simulink model "week2pro4"  (R2020b)
settings: Solver=VariableStepAuto  StartTime=0.0  StopTime=10.0  RelTol=1e-3
model workspace (MAT data in the model file):
  J = 3.224e-06
  K = 0.0274
  L = 2.75e-06
  R = 4
  b = 3.2577e-06
  kd = 0.14068535322
  ki = 523.295635458
  kp = 17.35894986
settings Model: Creator=admin  LastModifiedBy=admin

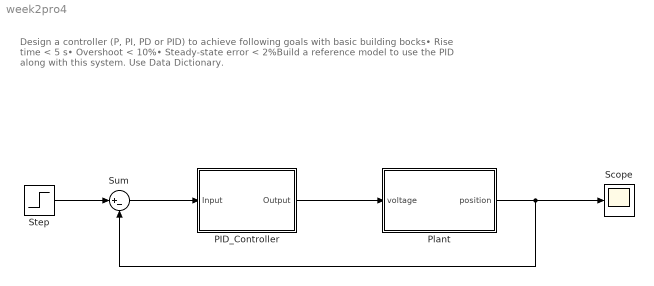
== system week2pro4 ==
  note: Design a controller (P, PI, PD or PID) to achieve following goals with basic building bocks• Rise time < 5 s• Overshoot < 10%• Steady-state error < 2%Build a reference model to use the PID along with this system. Use Data Dictionary.
  PID_Controller : Subsystem
  Plant : Subsystem
  Scope : Scope
  Step : Step  SampleTime=0
  Sum : Sum  Inputs=|+-
  wires:
  PID_Controller/1(Output) -> Plant/1(voltage)
  Sum/1 -> PID_Controller/1(Input)
  Step/1 -> Sum/1
  Plant/1(position) -> Sum/2, Scope/1

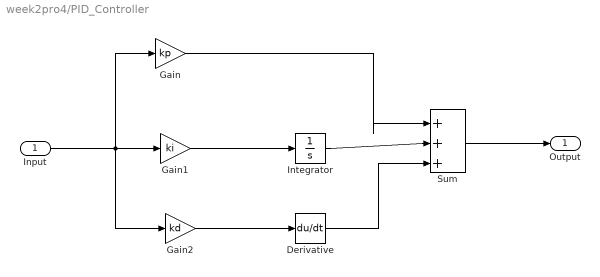
== system week2pro4/PID_Controller ==
  Input : Inport
  Derivative : Derivative
  Gain : Gain  Gain=kp
  Gain1 : Gain  Gain=ki
  Gain2 : Gain  Gain=kd
  Integrator : Integrator
  Sum : Sum  Inputs=|+++
  Output : Outport
  wires:
  Gain1/1 -> Integrator/1
  Input/1 -> Gain2/1, Gain/1, Gain1/1
  Derivative/1 -> Sum/3
  Gain/1 -> Sum/1
  Sum/1 -> Output/1
  Integrator/1 -> Sum/2
  Gain2/1 -> Derivative/1

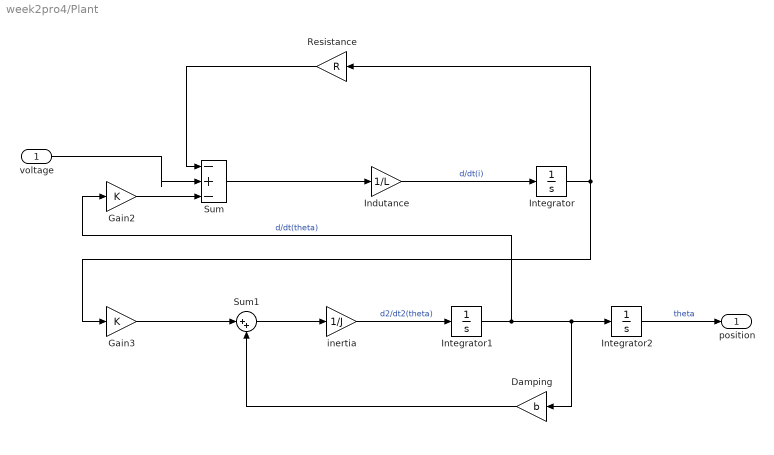
== system week2pro4/Plant ==
  voltage : Inport
  Damping : Gain  Gain=b
  Gain2 : Gain  Gain=K
  Gain3 : Gain  Gain=K
  Indutance : Gain  Gain=1/L
  Integrator : Integrator
  Integrator1 : Integrator
  Integrator2 : Integrator
  Resistance : Gain  Gain=R
  Sum : Sum  Inputs=|-+-
  Sum1 : Sum  Inputs=|++
  inertia : Gain  Gain=1/J
  position : Outport
  wires:
  Gain3/1 -> Sum1/1
  Gain2/1 -> Sum/3
  Resistance/1 -> Sum/1
  Sum1/1 -> inertia/1
  Integrator1/1 -> Gain2/1, Damping/1, Integrator2/1  "d/dt(theta)"
  voltage/1 -> Sum/2
  Integrator/1 -> Gain3/1, Resistance/1
  Indutance/1 -> Integrator/1  "d/dt(i)"
  Damping/1 -> Sum1/2
  inertia/1 -> Integrator1/1  "d2/dt2(theta)"
  Sum/1 -> Indutance/1
  Integrator2/1 -> position/1  "theta"
